simulink library "INT_InjCrv_PiI1"  (R2016b)
settings: Solver=VariableStepAuto  StartTime=0.0  StopTime=10.0  RelTol=1e-3
settings Model: Creator=mayongchao  LastModifiedBy=mayongchao

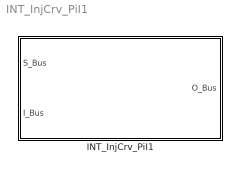
== system INT_InjCrv_PiI1 ==
  INT_InjCrv_PiI1 : Subsystem

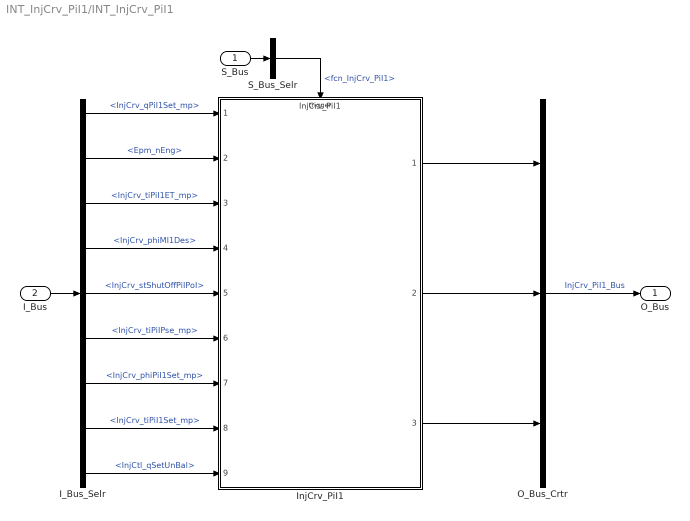
== system INT_InjCrv_PiI1/INT_InjCrv_PiI1 ==
  S_Bus : Inport
  I_Bus : Inport  Port=2
  I_Bus_Selr : BusSelector  OutputSignals=InjCrv_qPiI1Set_mp,Epm_nEng,InjCrv_tiPiI1ET_mp,InjCrv_phiMI1Des,InjCrv_stShutOffPiIPoI,InjCrv_tiPiIPse_mp,InjCrv_phiPiI1Set_mp,InjCrv_tiPiI1Set_mp,InjCtl_qSetUnBal
  InjCrv_PiI1 : ModelReference  ModelNameDialog=InjCrv_PiI1  SimulationMode=Normal  ModelReferenceVersion=1.28  TriggerPortName=function  TriggerPortTriggerType=function-call  TriggerPortStatesWhenEnabling=held
  O_Bus_Crtr : BusCreator  Inputs=3
  S_Bus_Selr : BusSelector  OutputSignals=fcn_InjCrv_PiI1
  O_Bus : Outport
  wires:
  S_Bus_Selr/1 -> InjCrv_PiI1/Trigger  "<fcn_InjCrv_PiI1>"
  S_Bus/1 -> S_Bus_Selr/1
  I_Bus/1 -> I_Bus_Selr/1
  I_Bus_Selr/1 -> InjCrv_PiI1/1  "<InjCrv_qPiI1Set_mp>"
  I_Bus_Selr/2 -> InjCrv_PiI1/2  "<Epm_nEng>"
  I_Bus_Selr/3 -> InjCrv_PiI1/3  "<InjCrv_tiPiI1ET_mp>"
  I_Bus_Selr/4 -> InjCrv_PiI1/4  "<InjCrv_phiMI1Des>"
  I_Bus_Selr/5 -> InjCrv_PiI1/5  "<InjCrv_stShutOffPiIPoI>"
  I_Bus_Selr/6 -> InjCrv_PiI1/6  "<InjCrv_tiPiIPse_mp>"
  I_Bus_Selr/7 -> InjCrv_PiI1/7  "<InjCrv_phiPiI1Set_mp>"
  I_Bus_Selr/8 -> InjCrv_PiI1/8  "<InjCrv_tiPiI1Set_mp>"
  I_Bus_Selr/9 -> InjCrv_PiI1/9  "<InjCtl_qSetUnBal>"
  O_Bus_Crtr/1 -> O_Bus/1  "InjCrv_PiI1_Bus"
  InjCrv_PiI1/1 -> O_Bus_Crtr/1
  InjCrv_PiI1/2 -> O_Bus_Crtr/2
  InjCrv_PiI1/3 -> O_Bus_Crtr/3
